simulink model "induction_foc"  (R2022b)
settings: Solver=ode15s  StartTime=0.0  StopTime=2  MaxStep=1e-4  MinStep=1e-7  RelTol=1e-3
values from neighbouring files (symbols this model uses):
  al = log(9)/tr_m    [parameters_4.m]
  as = log(9)/tr_s    [parameters_4.m]
  ba = 2 * K^2 * (as * J)/(3*np^2 * psi_nom)    [parameters_4.m]
  I_base = 3.6 * sqrt(2)    [parameters_4.m]
  Id_nom = psi_nom/LM    [parameters_4.m]
  J = 0.1    [parameters_4.m]
  J_m = J    (= 0.1)    [parameters_4.m]
  K = 1    [parameters_4.m]
  Ki = (ac^2)*Lsig    [parameters_4.m]
  Kis = 2*K^2 * as^2 * J/(3*np^2 * psi_nom)    [parameters_4.m]
  Kp = ac*Lsig    [parameters_4.m]
  Kps = 2*K^2 * as * J/(3*np^2 * psi_nom)    [parameters_4.m]
  ksi = (Lsig + LM)/Lsig    (= 10.2245098039)    [parameters_4.m]
  lamba = 1.5    [parameters_4.m]
  LM = b*Lm    (= 0.368980392157)    [parameters_4.m]
  LM_m = LM    (= 0.368980392157)    [parameters_4.m]
  LMest = LMest2    (= 0.368980392157)    [parameters_4.m]
  LMest2 = LM    (= 0.368980392157)    [parameters_4.m]
  Lsig = Lls+Llr    (= 0.04)    [parameters_4.m]
  Lsig_m = Lsig    (= 0.04)    [parameters_4.m]
  np = 2    [parameters_4.m]
  Ra = ac*Lsig-Rs-RR    [parameters_4.m]
  RR = (b^2)*Rr    (= 2.26090926567)    [parameters_4.m]
  RR_m = RR    (= 2.26090926567)    [parameters_4.m]
  RRest = RRest2    (= 2.26090926567)    [parameters_4.m]
  RRest2 = RR    (= 2.26090926567)    [parameters_4.m]
  Rs = 6.5    [parameters_4.m]
  Rs_m = Rs    (= 6.5)    [parameters_4.m]
  V_base = 60    [parameters_4.m]
  Vpeak = V_base    (= 60)    [parameters_4.m]
  w_base = 2*pi*50    (= 314.159265359)    [parameters_4.m]
  w_delta = 0.1*w_base    (= 31.4159265359)    [parameters_4.m]
undefined symbols (not defined in the file or in its folder): I_max, sigbuilder_block
libraries: simulink x2
settings Model: Creator=alexa  LastModifiedBy=alexa
settings SolverCC: InitialStep=1e-6

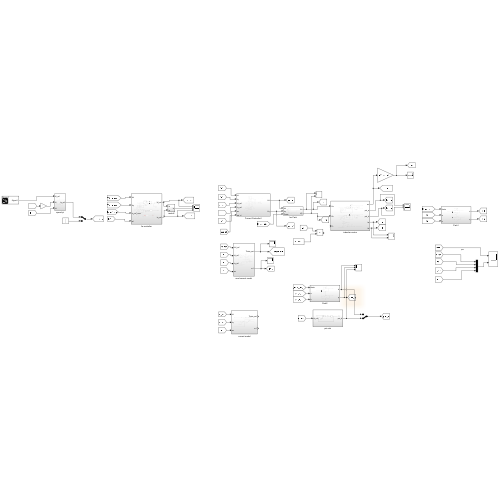
[thumbnail: Simulink's stored preview of the top-level diagram]
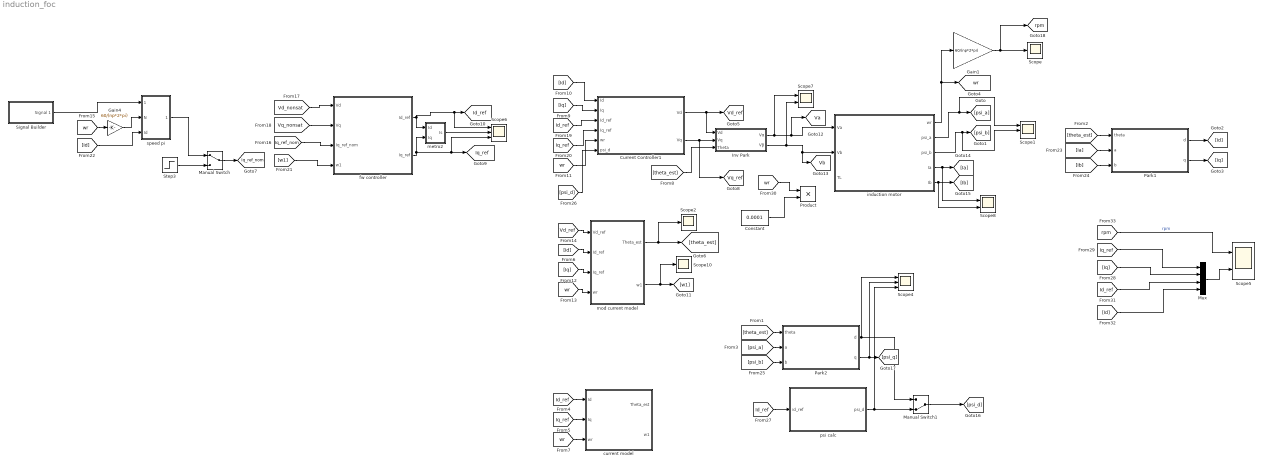
== system induction_foc ==
  Constant : Constant  Value=0.0001
  Current Controller1 : Subsystem
  Gain1 : Gain  Gain=60/(np*2*pi)
  Gain4 : Gain  Gain=60/(np*2*pi)
  Inv Park : Subsystem
  Manual Switch : ManualSwitch
  Manual Switch1 : ManualSwitch  CurrentSetting=0
  Mux : Mux
  Park1 : Subsystem
  Park2 : Subsystem
  Product : Product
  Scope : Scope
  Scope1 : Scope  NumInputPorts=3
  Scope10 : Scope
  Scope2 : Scope
  Scope4 : Scope  NumInputPorts=3
  Scope5 : Scope  NumInputPorts=2
  Scope6 : Scope  NumInputPorts=3
  Scope7 : Scope  NumInputPorts=2
  Scope8 : Scope  NumInputPorts=2
  Signal Builder : Subsystem  Tag=STV Subsys  LoadFcn=sigbuilder_block('load');  StartFcn=sigbuilder_block('start');  StopFcn=sigbuilder_block('stop');  ClipboardFcn=sigbuilder_block('clipboard');  mask(Sigbuilder block){tuvar=[0:10]}
      mask help: Simulink:masks:SigbuilderBlock_MD
      mask init:
      | if ~strcmp(get_param(bdroot(gcbh),'SimulationStatus'),'stopped') tuvar = sigbuilder_block('maskInit'); end
      settings: CopyFcn=sigbuilder_block('copy');  DeleteFcn=sigbuilder_block('delete');  ModelCloseFcn=sigbuilder_block('modelClose');  PreSaveFcn=sigbuilder_block('preSave');  PauseFcn=sigbuilder_block('pause');  ContinueFcn=sigbuilder_block('continue');  NameChangeFcn=sigbuilder_block('namechange');  OpenFcn=sigbuilder_block('open',[437.6 199.2 550.4 400 ]);  CloseFcn=sigbuilder_block('close');
      mask Display: plot(0, 0, 100, 100,[2, 2, 32, 32, 2], [68, 8, 8, 68, 68],[32, 2], [38, 38], [32, 19, 2],[53, 60, 44], [32, 17, 17, 2],[16, 16, 31, 31]);txt = getActiveGroup(gcbh);text(2, 100, txt,'verticalAlignment', 'top');
  Step3 : Step  Time=0.3  After=3  SampleTime=0
  current model : Subsystem
  fw controller : Subsystem
  induction motor : Subsystem
  metro2 : Subsystem
  mod current model : Subsystem
  psi calc : Subsystem
  speed pi : Subsystem
  tag scope: Id_ref=global, Iq_ref=global, Iq_ref_nom=global, Va=global, Vb=global, Vd_ref=global, Vq_ref=global, rpm=global, wr=global
  wires:
  Inv Park/1(Vα) -> Scope7/1, [Va], induction motor/1(Va)
  Inv Park/2(Vβ) -> Scope7/2, [Vb], induction motor/2(Vb)
  induction motor/1(wr) -> Gain1/1, [wr]
  induction motor/2(psi_a) -> Scope1/1, [psi_a]
  induction motor/3(psi_b) -> Scope1/2, [psi_b]
  [theta_est] -> Park1/1(theta)
  Park1/1(d) -> [Id]
  Park1/2(q) -> [Iq]
  Current Controller1/2(Vq) -> [Vq_ref], Inv Park/2(Vq)
  Current Controller1/1(Vd) -> [Vd_ref], Inv Park/1(Vd)
  [theta_est] -> Inv Park/3(Theta)
  [Id_ref] -> Current Controller1/3(Id_ref)
  [Iq] -> Current Controller1/2(Iq)
  [Id] -> Current Controller1/1(Id)
  [wr] -> Current Controller1/5(wr)
  Gain4/1 -> speed pi/2(N)
  Signal Builder/1(Signal 1) -> speed pi/1(N_ref)
  [Id_ref] -> current model/1(Id)
  [wr] -> current model/3(wr)
  [Iq_ref] -> current model/2(Iq)
  [Iq] -> mod current model/3(Iq_ref)
  [Id] -> mod current model/2(Id_ref)
  [wr] -> mod current model/4(wr)
  [Vd_ref] -> mod current model/1(Vd_ref)
  [wr] -> Gain4/1
  [Vd_nonsat] -> fw controller/1(Vd)
  [Vq_nonsat] -> fw controller/2(Vq)
  [Iq_ref] -> Current Controller1/4(Iq_ref)
  fw controller/2(Iq_ref) -> metro2/2(Iq), Scope6/3, [Iq_ref]
  fw controller/1(Id_ref) -> Scope6/1, [Id_ref], metro2/1(Id)
  [w1] -> fw controller/4(w1)
  Gain1/1 -> [rpm], Scope/1
  metro2/1(Is) -> Scope6/2
  [Iq_ref_nom] -> fw controller/3(Iq_ref_nom)
  [Id] -> speed pi/3(Id)
  mod current model/1(Theta_est) -> Scope2/1, [theta_est]
  mod current model/2(w1) -> Scope10/1, [w1]
  induction motor/4(Ia) -> Scope8/1, [Ia]
  induction motor/5(Ib) -> Scope8/2, [Ib]
  [Ib] -> Park1/3(b)
  [Ia] -> Park1/2(a)
  [theta_est] -> Park2/1(theta)
  [psi_a] -> Park2/2(a)
  [psi_b] -> Park2/3(b)
  Park2/1(d) -> Scope4/1, Manual Switch1/1
  Park2/2(q) -> Scope4/2, [psi_q]
  [psi_d] -> Current Controller1/6(psi_d)
  psi calc/1(psi_d) -> Manual Switch1/2, Scope4/3
  [Id_ref] -> psi calc/1(id_ref)
  [wr] -> Product/1
  Constant/1 -> Product/2
  Step3/1 -> Manual Switch/2
  speed pi/1(Iq_ref) -> Manual Switch/1
  Manual Switch/1 -> [Iq_ref_nom]
  Manual Switch1/1 -> [psi_d]
  [Iq_ref] -> Mux/1
  [Iq] -> Mux/2
  [Id_ref] -> Mux/3
  [Id] -> Mux/4
  Mux/1 -> Scope5/2
  [rpm] -> Scope5/1  "rpm"

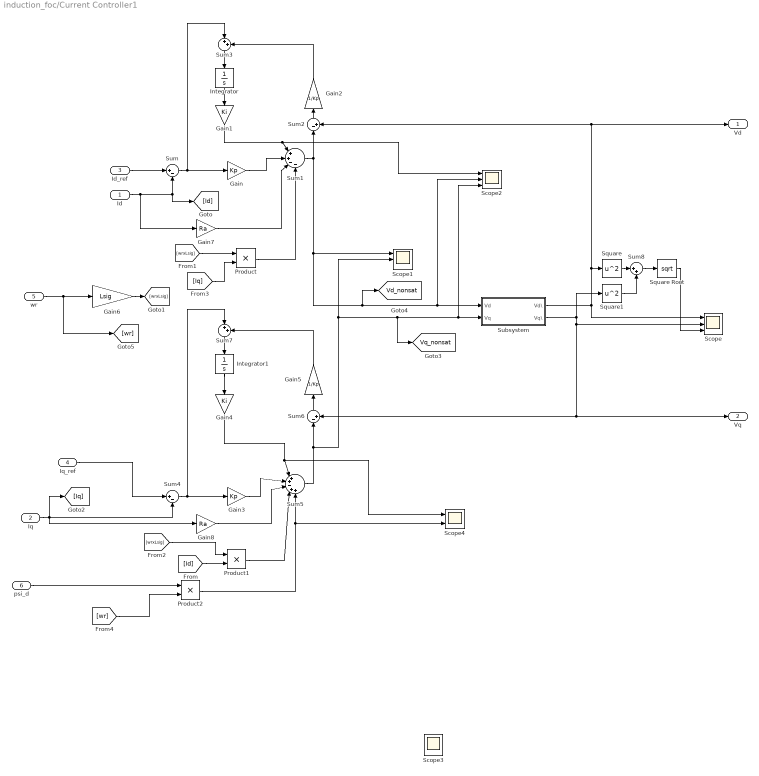
== system induction_foc/Current Controller1 ==
  Id : Inport
  Iq : Inport  Port=2
  Id_ref : Inport  Port=3
  Iq_ref : Inport  Port=4
  wr : Inport  Port=5
  psi_d : Inport  Port=6
  Gain : Gain  Gain=Kp
  Gain1 : Gain  Gain=Ki
  Gain2 : Gain  Gain=1/Kp
  Gain3 : Gain  Gain=Kp
  Gain4 : Gain  Gain=Ki
  Gain5 : Gain  Gain=1/Kp
  Gain6 : Gain  Gain=Lsig
  Gain7 : Gain  Gain=Ra
  Gain8 : Gain  Gain=Ra
  Integrator : Integrator
  Integrator1 : Integrator
  Product : Product
  Product1 : Product
  Product2 : Product
  Scope{,1..3} (4 alike) : Scope  NumInputPorts=3
  Scope4 : Scope  NumInputPorts=2
  Square : Math  Operator=square
  Square Root : Sqrt
  Square1 : Math  Operator=square
  Subsystem : Subsystem
  Sum : Sum  Inputs=|+-
  Sum1 : Sum  Inputs=|++--
  Sum2 : Sum  Inputs=|-+
  Sum3 : Sum  Inputs=|++
  Sum4 : Sum  Inputs=|+-
  Sum5 : Sum  Inputs=|++-++
  Sum6 : Sum  Inputs=|-+
  Sum7 : Sum  Inputs=|++
  Sum8 : Sum  Inputs=|++
  Vd : Outport
  Vq : Outport  Port=2
  tag scope: Vd_nonsat=global, Vq_nonsat=global
  wires:
  Id_ref/1 -> Sum/1
  Id/1 -> Gain7/1, [Id], Sum/2
  Sum/1 -> Sum3/1, Gain/1
  Subsystem/1(Vd\) -> Square/1, Sum2/2, Vd/1, Scope/1
  Integrator/1 -> Gain1/1
  Sum3/1 -> Integrator/1
  Sum2/1 -> Gain2/1
  Gain/1 -> Sum1/2
  Gain1/1 -> Scope2/1, Sum1/1
  Gain5/1 -> Sum7/2
  Integrator1/1 -> Gain4/1
  Sum4/1 -> Sum7/1, Gain3/1
  Subsystem/2(Vq\) -> Scope/2, Sum6/2, Vq/1, Square1/1
  Gain3/1 -> Sum5/2
  Gain4/1 -> Scope4/1, Sum5/1
  Sum7/1 -> Integrator1/1
  Iq_ref/1 -> Sum4/1
  Sum6/1 -> Gain5/1
  Sum5/1 -> Sum6/1, [Vq_nonsat], Scope2/3, Subsystem/2(Vq), Scope1/2
  Iq/1 -> Gain8/1, Sum4/2, [Iq]
  wr/1 -> [wr], Gain6/1
  Product/1 -> Sum1/4
  [Id] -> Product1/2
  Gain6/1 -> [wrxLsig]
  [wrxLsig] -> Product/1
  [wrxLsig] -> Product1/1
  Product1/1 -> Sum5/4
  [Iq] -> Product/2
  Gain7/1 -> Sum1/3
  Gain8/1 -> Sum5/3
  Gain2/1 -> Sum3/2
  Square/1 -> Sum8/1
  Square1/1 -> Sum8/2
  Sum8/1 -> Square Root/1
  Square Root/1 -> Scope/3
  Sum1/1 -> [Vd_nonsat], Scope2/2, Subsystem/1(Vd), Scope1/1, Sum2/1
  psi_d/1 -> Product2/1
  [wr] -> Product2/2
  Product2/1 -> Scope4/2, Sum5/5

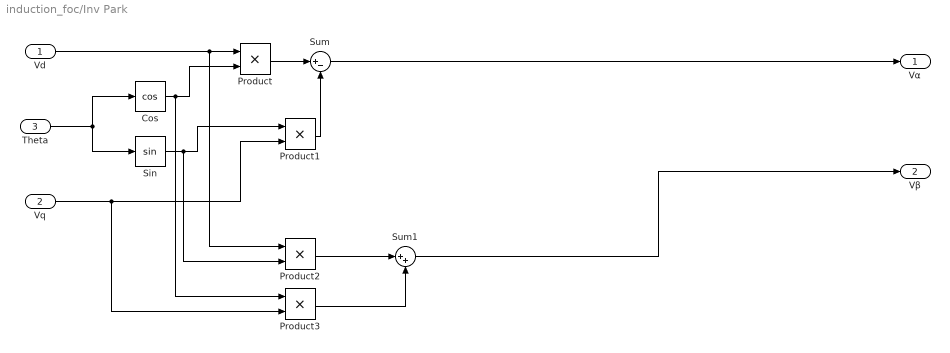
== system induction_foc/Inv Park ==
  Vd : Inport
  Vq : Inport  Port=2
  Theta : Inport  Port=3
  Cos : Trigonometry  Operator=cos
  Product{,1..3} (4 alike) : Product
  Sin : Trigonometry
  Sum : Sum  Inputs=|+-
  Sum1 : Sum  Inputs=|++
  Vα : Outport
  Vβ : Outport  Port=2
  wires:
  Theta/1 -> Sin/1, Cos/1
  Vd/1 -> Product2/1, Product/1
  Cos/1 -> Product3/1, Product/2
  Product/1 -> Sum/1
  Sin/1 -> Product2/2, Product1/1
  Vq/1 -> Product3/2, Product1/2
  Product1/1 -> Sum/2
  Sum/1 -> Vα/1
  Product2/1 -> Sum1/1
  Product3/1 -> Sum1/2
  Sum1/1 -> Vβ/1

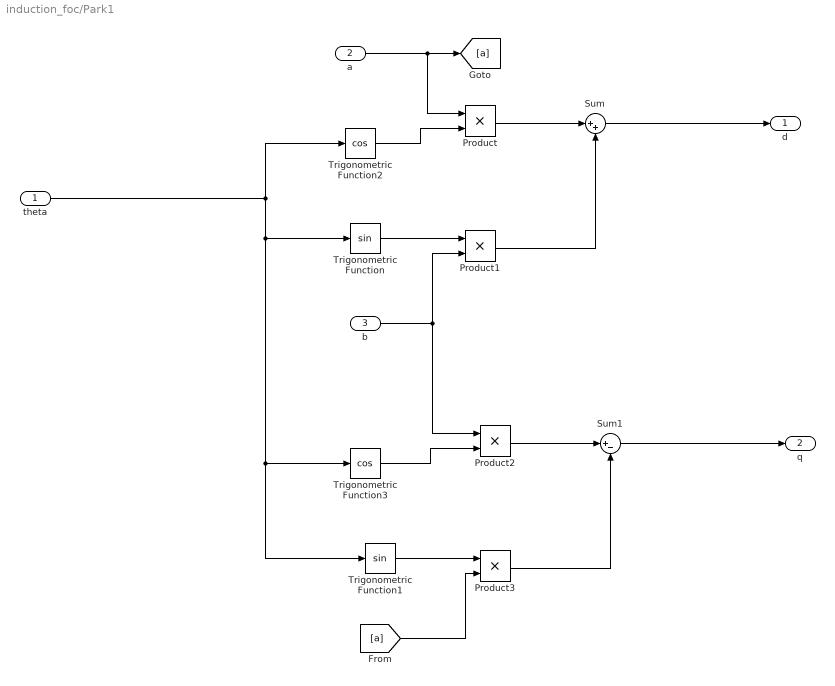
== system induction_foc/Park1 ==
  theta : Inport
  a : Inport  Port=2
  b : Inport  Port=3
  Product{,1..3} (4 alike) : Product
  Sum : Sum  Inputs=|++
  Sum1 : Sum  Inputs=|+-
  Trigonometric Function : Trigonometry
  Trigonometric Function1 : Trigonometry
  Trigonometric Function2 : Trigonometry  Operator=cos
  Trigonometric Function3 : Trigonometry  Operator=cos
  d : Outport
  q : Outport  Port=2
  wires:
  Trigonometric Function2/1 -> Product/2
  a/1 -> [a], Product/1
  Product/1 -> Sum/1
  Trigonometric Function/1 -> Product1/1
  b/1 -> Product1/2, Product2/1
  Product1/1 -> Sum/2
  Sum/1 -> d/1
  Trigonometric Function3/1 -> Product2/2
  Trigonometric Function1/1 -> Product3/1
  Sum1/1 -> q/1
  Product2/1 -> Sum1/1
  Product3/1 -> Sum1/2
  [a] -> Product3/2
  theta/1 -> Trigonometric Function/1, Trigonometric Function3/1, Trigonometric Function1/1, Trigonometric Function2/1

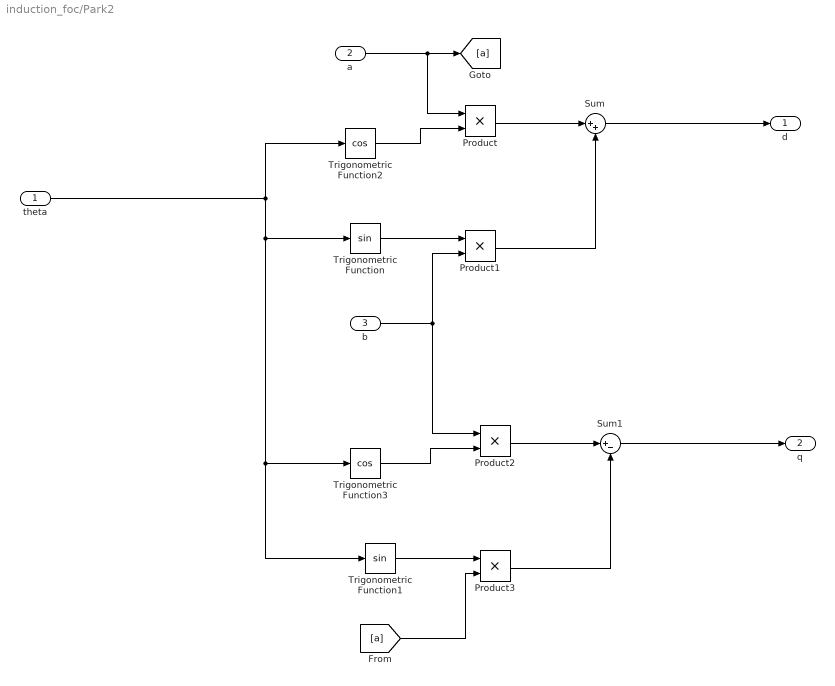
== system induction_foc/Park2 ==
  theta : Inport
  a : Inport  Port=2
  b : Inport  Port=3
  Product{,1..3} (4 alike) : Product
  Sum : Sum  Inputs=|++
  Sum1 : Sum  Inputs=|+-
  Trigonometric Function : Trigonometry
  Trigonometric Function1 : Trigonometry
  Trigonometric Function2 : Trigonometry  Operator=cos
  Trigonometric Function3 : Trigonometry  Operator=cos
  d : Outport
  q : Outport  Port=2
  wires:
  Trigonometric Function2/1 -> Product/2
  a/1 -> [a], Product/1
  Product/1 -> Sum/1
  Trigonometric Function/1 -> Product1/1
  b/1 -> Product1/2, Product2/1
  Product1/1 -> Sum/2
  Sum/1 -> d/1
  Trigonometric Function3/1 -> Product2/2
  Trigonometric Function1/1 -> Product3/1
  Sum1/1 -> q/1
  Product2/1 -> Sum1/1
  Product3/1 -> Sum1/2
  [a] -> Product3/2
  theta/1 -> Trigonometric Function/1, Trigonometric Function3/1, Trigonometric Function1/1, Trigonometric Function2/1

== system induction_foc/Signal Builder ==
  Demux : Demux  Tag=STV Demux  Outputs=1
      settings: DisplayOption=none
  FromWs : FromWorkspace  Tag=STV FromWs  VariableName=tuvar
      SigBuilderData=|
      | common.afterFinalStr = 'Extrapolate'
      | common.sampleTime = 0
      | dataSet.timeRange = [0 10]
      | dataSet.name = 'Group 1'
      | sbobj.Groups.Name = 'Group 1'
      | sbobj.Groups.Signals.Name = 'Signal 1'
      | sbobj.Groups.Signals.XData = [0 0.5 0.5 1 1 10]
      | sbobj.Groups.Signals.YData = [0 52 200 200 0 0]
  Signal 1 : Outport  Tag=STV Outport
  wires:
  Demux/1 -> Signal 1/1
  FromWs/1 -> Demux/1

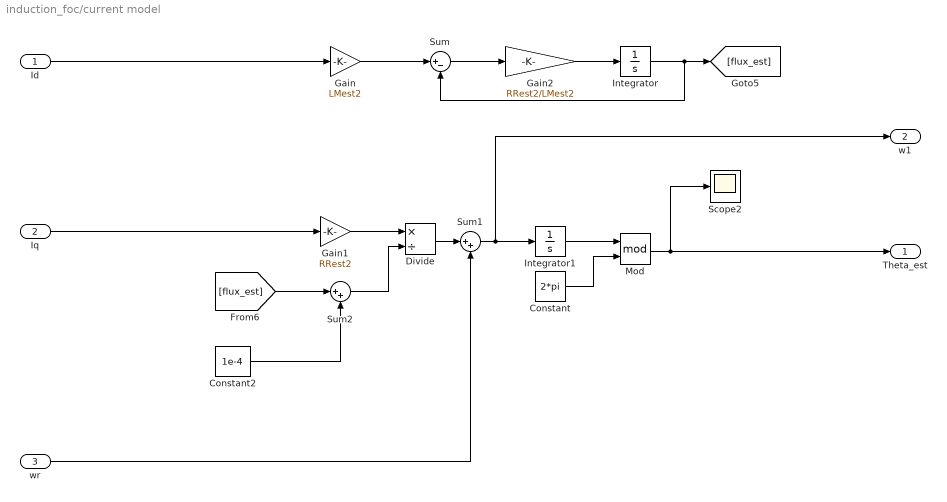
== system induction_foc/current model ==
  Id : Inport
  Iq : Inport  Port=2
  wr : Inport  Port=3
  Constant : Constant  Value=2*pi
  Constant2 : Constant  Value=1e-4
  Divide : Product  Inputs=*/
  Gain : Gain  Gain=LMest2
  Gain1 : Gain  Gain=RRest2
  Gain2 : Gain  Gain=RRest2/LMest2
  Integrator : Integrator
  Integrator1 : Integrator
  Mod : Math  Operator=mod
  Scope2 : Scope
  Sum : Sum  Inputs=|+-
  Sum1 : Sum  Inputs=|++
  Sum2 : Sum  Inputs=|++
  Theta_est : Outport
  w1 : Outport  Port=2
  wires:
  Sum2/1 -> Divide/2
  Constant/1 -> Mod/2
  Integrator/1 -> Sum/2, [flux_est]
  Divide/1 -> Sum1/1
  Gain/1 -> Sum/1
  [flux_est] -> Sum2/1
  Constant2/1 -> Sum2/2
  Sum1/1 -> w1/1, Integrator1/1
  wr/1 -> Sum1/2
  Gain1/1 -> Divide/1
  Gain2/1 -> Integrator/1
  Id/1 -> Gain/1
  Sum/1 -> Gain2/1
  Mod/1 -> Theta_est/1, Scope2/1
  Iq/1 -> Gain1/1
  Integrator1/1 -> Mod/1

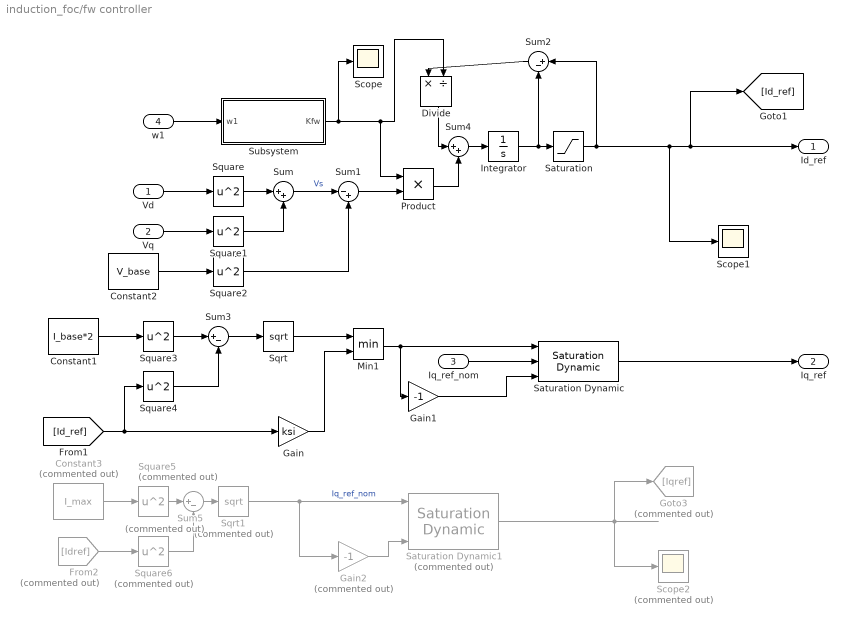
== system induction_foc/fw controller ==
  Vd : Inport
  Vq : Inport  Port=2
  Iq_ref_nom : Inport  Port=3
  w1 : Inport  Port=4
  Constant1 : Constant  Value=I_base*2
  Constant2 : Constant  Value=V_base
  Constant3 : Constant  Commented=on  Value=I_max
  Divide : Product  Inputs=*/
  From2 : From  Commented=on  GotoTag=Idref
  Gain : Gain  Gain=ksi
  Gain1 : Gain  Gain=-1
  Gain2 : Gain  Commented=on  Gain=-1
  Goto3 : Goto  Commented=on  GotoTag=Iqref
  Integrator : Integrator
  Min1 : MinMax  Inputs=2
  Product : Product
  Saturation : Saturate  UpperLimit=Id_nom  LowerLimit=0.05*Id_nom
  Saturation Dynamic : simulink/Discontinuities/Saturation Dynamic  OutMin=[]  OutMax=[]  OutDataTypeStr=Inherit: Same as second input  OutDataType=fixdt(1, 16)  OutScaling=2^-10  DoSatur=off
  Saturation Dynamic1 : simulink/Discontinuities/Saturation Dynamic  Commented=on  OutMin=[]  OutMax=[]  OutDataTypeStr=Inherit: Same as second input  OutDataType=fixdt(1, 16)  OutScaling=2^-10  DoSatur=off
  Scope : Scope
  Scope1 : Scope
  Scope2 : Scope  Commented=on
  Sqrt : Sqrt
  Sqrt1 : Sqrt  Commented=on
  Square{,1..4} (5 alike) : Math  Operator=square
  Square5 : Math  Commented=on  Operator=square
  Square6 : Math  Commented=on  Operator=square
  Subsystem : Subsystem
  Sum : Sum  Inputs=|++
  Sum1 : Sum  Inputs=|-+
  Sum2 : Sum  Inputs=|+-
  Sum3 : Sum  Inputs=|+-
  Sum4 : Sum  Inputs=|++
  Sum5 : Sum  Commented=on  Inputs=|+-
  Id_ref : Outport
  Iq_ref : Outport  Port=2
  wires:
  Vd/1 -> Square/1
  Vq/1 -> Square1/1
  Constant2/1 -> Square2/1
  Square/1 -> Sum/1
  Square1/1 -> Sum/2
  Sum/1 -> Sum1/1  "Vs"
  Square2/1 -> Sum1/2
  Sum1/1 -> Product/2
  Integrator/1 -> Sum2/2, Saturation/1
  w1/1 -> Subsystem/1(w1)
  Subsystem/1(Kfw) -> Scope/1, Divide/2, Product/1
  Constant1/1 -> Square3/1
  Square3/1 -> Sum3/1
  Square4/1 -> Sum3/2
  Sum3/1 -> Sqrt/1
  Sqrt/1 -> Min1/1
  Gain/1 -> Min1/2
  [Id_ref] -> Square4/1, Gain/1
  Iq_ref_nom/1 -> Saturation Dynamic/2
  Min1/1 -> Gain1/1, Saturation Dynamic/1
  Gain1/1 -> Saturation Dynamic/3
  Saturation Dynamic/1 -> Iq_ref/1
  Saturation/1 -> Sum2/1, Scope1/1, [Id_ref], Id_ref/1
  Product/1 -> Sum4/2
  Sum4/1 -> Integrator/1
  Sum2/1 -> Divide/1
  Divide/1 -> Sum4/1
  ? -> Saturation Dynamic1/2
  Sum5/1 -> Sqrt1/1
  Square6/1 -> Sum5/2
  From2/1 -> Square6/1
  Saturation Dynamic1/1 -> Scope2/1, Goto3/1
  Square5/1 -> Sum5/1
  Sqrt1/1 -> Saturation Dynamic1/1, Gain2/1  "Iq_ref_nom"
  Constant3/1 -> Square5/1
  Gain2/1 -> Saturation Dynamic1/3

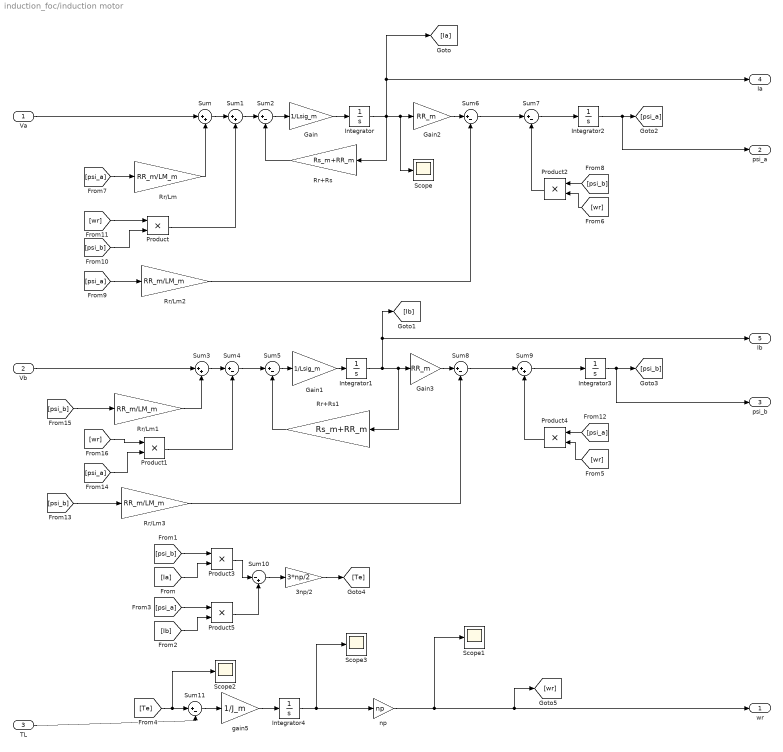
== system induction_foc/induction motor ==
  Va : Inport
  Vb : Inport  Port=2
  TL : Inport  Port=3
  3np/2 : Gain  Gain=3*np/2
  Gain : Gain  Gain=1/Lsig_m
  Gain1 : Gain  Gain=1/Lsig_m
  Gain2 : Gain  Gain=RR_m
  Gain3 : Gain  Gain=RR_m
  Integrator{,1..4} (5 alike) : Integrator
  Product{,1..5} (6 alike) : Product
  Rr+Rs : Gain  Gain=Rs_m+RR_m
  Rr+Rs1 : Gain  Gain=Rs_m+RR_m
  Rr/Lm{,1..3} (4 alike) : Gain  Gain=RR_m/LM_m
  Scope{,1..3} (4 alike) : Scope
  Sum{,1,3,9} (4 alike) : Sum  Inputs=|++
  Sum10 : Sum  Inputs=|-+
  Sum{2,4..8,11} (7 alike) : Sum  Inputs=|+-
  gain5 : Gain  Gain=1/J_m
  np : Gain  Gain=np
  wr : Outport
  psi_a : Outport  Port=2
  psi_b : Outport  Port=3
  Ia : Outport  Port=4
  Ib : Outport  Port=5
  wires:
  Va/1 -> Sum/1
  Sum/1 -> Sum1/1
  Rr/Lm/1 -> Sum/2
  Integrator2/1 -> psi_a/1, [psi_a]
  Product/1 -> Sum1/2
  Rr+Rs/1 -> Sum2/2
  Integrator/1 -> Scope/1, Gain2/1, Ia/1, [Ia], Rr+Rs/1
  Sum1/1 -> Sum2/1
  Sum2/1 -> Gain/1
  Gain/1 -> Integrator/1
  Integrator3/1 -> psi_b/1, [psi_b]
  Gain1/1 -> Integrator1/1
  Sum4/1 -> Sum5/1
  Integrator1/1 -> Rr+Rs1/1, Gain3/1, [Ib], Ib/1
  Sum5/1 -> Gain1/1
  Vb/1 -> Sum3/1
  Sum3/1 -> Sum4/1
  Rr+Rs1/1 -> Sum5/2
  Product1/1 -> Sum4/2
  Gain2/1 -> Sum6/1
  Rr/Lm2/1 -> Sum6/2
  Sum6/1 -> Sum7/1
  Product2/1 -> Sum7/2
  Sum7/1 -> Integrator2/1
  Rr/Lm3/1 -> Sum8/2
  Product4/1 -> Sum9/2
  Sum8/1 -> Sum9/1
  Sum9/1 -> Integrator3/1
  Gain3/1 -> Sum8/1
  [psi_b] -> Product3/1
  [Ia] -> Product3/2
  [psi_a] -> Product5/1
  [Ib] -> Product5/2
  Product3/1 -> Sum10/1
  Product5/1 -> Sum10/2
  Sum10/1 -> 3np/2/1
  3np/2/1 -> [Te]
  [Te] -> Scope2/1, Sum11/1
  Sum11/1 -> gain5/1
  gain5/1 -> Integrator4/1
  TL/1 -> Sum11/2
  [wr] -> Product4/2
  np/1 -> Scope1/1, [wr], wr/1
  [psi_a] -> Rr/Lm/1
  [psi_b] -> Product2/1
  [wr] -> Product2/2
  [psi_a] -> Rr/Lm2/1
  [psi_b] -> Product/2
  [wr] -> Product/1
  [psi_a] -> Product4/1
  [psi_a] -> Product1/2
  [psi_b] -> Rr/Lm1/1
  [wr] -> Product1/1
  Integrator4/1 -> Scope3/1, np/1
  Rr/Lm1/1 -> Sum3/2
  [psi_b] -> Rr/Lm3/1

== system induction_foc/metro2 ==
  Id : Inport
  Iq : Inport  Port=2
  Sqrt : Sqrt
  Square : Math  Operator=square
  Square1 : Math  Operator=square
  Sum : Sum  Inputs=|++
  Is : Outport
  wires:
  Id/1 -> Square/1
  Iq/1 -> Square1/1
  Square/1 -> Sum/1
  Square1/1 -> Sum/2
  Sum/1 -> Sqrt/1
  Sqrt/1 -> Is/1

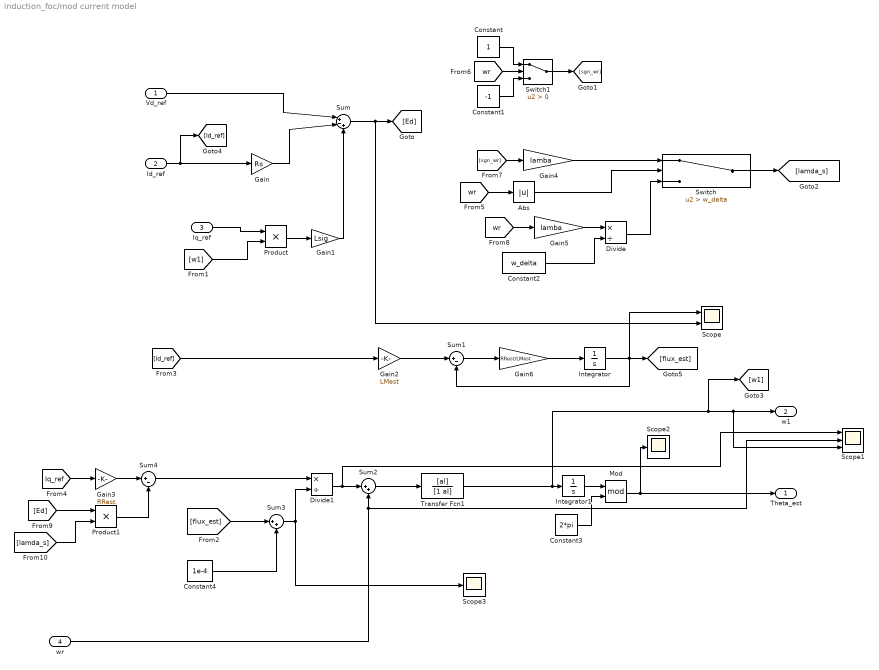
== system induction_foc/mod current model ==
  Vd_ref : Inport
  Id_ref : Inport  Port=2
  Iq_ref : Inport  Port=3
  wr : Inport  Port=4
  Abs : Abs  SaturateOnIntegerOverflow=off
  Constant : Constant
  Constant1 : Constant  Value=-1
  Constant2 : Constant  Value=w_delta
  Constant3 : Constant  Value=2*pi
  Constant4 : Constant  Value=1e-4
  Divide : Product  Inputs=*/
  Divide1 : Product  Inputs=*/
  Gain : Gain  Gain=Rs
  Gain1 : Gain  Gain=Lsig
  Gain2 : Gain  Gain=LMest
  Gain3 : Gain  Gain=RRest
  Gain4 : Gain  Gain=lamba
  Gain5 : Gain  Gain=lamba
  Gain6 : Gain  Gain=RRest/LMest
  Integrator : Integrator
  Integrator1 : Integrator
  Mod : Math  Operator=mod
  Product : Product
  Product1 : Product
  Scope : Scope  NumInputPorts=2
  Scope1 : Scope  NumInputPorts=3
  Scope2 : Scope
  Scope3 : Scope
  Sum : Sum  Inputs=|+-+
  Sum1 : Sum  Inputs=|+-
  Sum2 : Sum  Inputs=|++
  Sum3 : Sum  Inputs=|++
  Sum4 : Sum  Inputs=|+-
  Switch : Switch  Criteria=u2 > Threshold  Threshold=w_delta  SaturateOnIntegerOverflow=off  InputSameDT=off
  Switch1 : Switch  Criteria=u2 > Threshold  SaturateOnIntegerOverflow=off  InputSameDT=off
  Transfer Fcn1 : TransferFcn  Numerator=[al]  Denominator=[1 al]
  Theta_est : Outport
  w1 : Outport  Port=2
  wires:
  Vd_ref/1 -> Sum/1
  Gain/1 -> Sum/2
  [w1] -> Product/2
  Product/1 -> Gain1/1
  Gain1/1 -> Sum/3
  Sum/1 -> Scope/2, [Ed]
  [wr] -> Abs/1
  Abs/1 -> Switch/2
  [wr] -> Switch1/2
  Constant/1 -> Switch1/1
  Constant1/1 -> Switch1/3
  Switch1/1 -> [sgn_wr]
  [sgn_wr] -> Gain4/1
  Gain4/1 -> Switch/1
  [wr] -> Gain5/1
  Gain5/1 -> Divide/1
  Constant2/1 -> Divide/2
  Divide/1 -> Switch/3
  Switch/1 -> [lamda_s]
  Id_ref/1 -> [Id_ref], Gain/1
  Iq_ref/1 -> Product/1
  Constant4/1 -> Sum3/2
  wr/1 -> Scope1/2, Sum2/2
  [flux_est] -> Sum3/1
  Gain6/1 -> Integrator/1
  Sum1/1 -> Gain6/1
  Integrator1/1 -> Mod/1
  Gain2/1 -> Sum1/1
  Mod/1 -> Scope2/1, Theta_est/1
  Divide1/1 -> Scope1/1, Sum2/1
  [Id_ref] -> Gain2/1
  Integrator/1 -> Sum1/2, Scope/1, [flux_est]
  Constant3/1 -> Mod/2
  Sum3/1 -> Divide1/2, Scope3/1
  [Iq_ref] -> Gain3/1
  Gain3/1 -> Sum4/1
  Sum4/1 -> Divide1/1
  Product1/1 -> Sum4/2
  [Ed] -> Product1/1
  [lamda_s] -> Product1/2
  Sum2/1 -> Transfer Fcn1/1
  Transfer Fcn1/1 -> [w1], Scope1/3, w1/1, Integrator1/1

== system induction_foc/psi calc ==
  id_ref : Inport
  Add : Sum  Inputs=+-
  Gain : Gain  Gain=1/LM
  Gain1 : Gain  Gain=RR
  Integrator : Integrator
  psi_d : Outport
  wires:
  id_ref/1 -> Add/1
  Add/1 -> Gain1/1
  Gain/1 -> Add/2
  Integrator/1 -> psi_d/1, Gain/1
  Gain1/1 -> Integrator/1

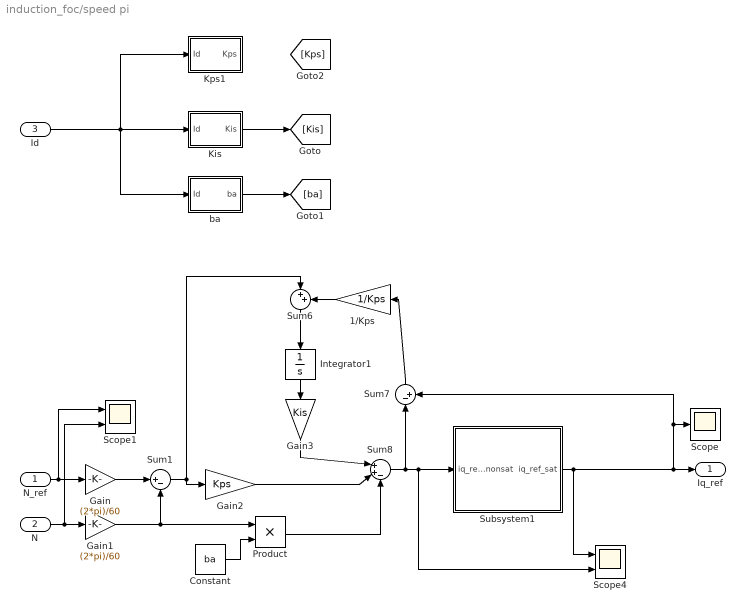
== system induction_foc/speed pi ==
  N_ref : Inport
  N : Inport  Port=2
  Id : Inport  Port=3
  1/Kps : Gain  Gain=1/Kps
  Constant : Constant  Value=ba
  Gain : Gain  Gain=(2*pi)/60
  Gain1 : Gain  Gain=(2*pi)/60
  Gain2 : Gain  Gain=Kps
  Gain3 : Gain  Gain=Kis
  Integrator1 : Integrator
  Kis : Subsystem
  Kps1 : Subsystem
  Product : Product
  Scope : Scope
  Scope1 : Scope  NumInputPorts=2
  Scope4 : Scope  NumInputPorts=2
  Subsystem1 : Subsystem
  Sum1 : Sum  Inputs=|+-
  Sum6 : Sum  Inputs=|++
  Sum7 : Sum  Inputs=|-+
  Sum8 : Sum  Inputs=|++-
  ba : Subsystem
  Iq_ref : Outport
  wires:
  Subsystem1/1(iq_ref_sat) -> Scope4/1, Sum7/2, Scope/1, Iq_ref/1
  Sum7/1 -> 1/Kps/1
  Sum8/1 -> Scope4/2, Subsystem1/1(iq_ref_nonsat), Sum7/1
  Gain2/1 -> Sum8/2
  1/Kps/1 -> Sum6/2
  Sum1/1 -> Gain2/1, Sum6/1
  N_ref/1 -> Scope1/1, Gain/1
  N/1 -> Scope1/2, Gain1/1
  Constant/1 -> Product/2
  Sum6/1 -> Integrator1/1
  Gain3/1 -> Sum8/1
  Product/1 -> Sum8/3
  Gain/1 -> Sum1/1
  Gain1/1 -> Product/1, Sum1/2
  Id/1 -> Kps1/1(Id), ba/1(Id), Kis/1(Id)
  Kis/1(Kis) -> [Kis]
  ba/1(ba) -> [ba]
  Integrator1/1 -> Gain3/1

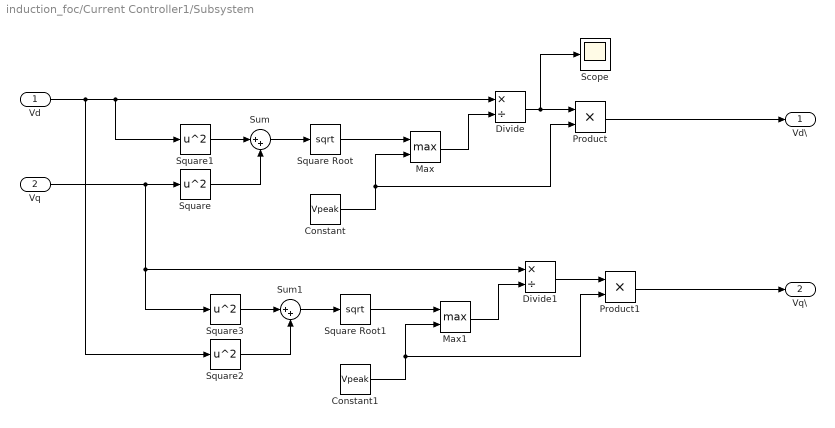
== system induction_foc/Current Controller1/Subsystem ==
  Vd : Inport
  Vq : Inport  Port=2
  Constant : Constant  Value=Vpeak
  Constant1 : Constant  Value=Vpeak
  Divide : Product  Inputs=*/
  Divide1 : Product  Inputs=*/
  Max : MinMax  Function=max  Inputs=2
  Max1 : MinMax  Function=max  Inputs=2
  Product : Product
  Product1 : Product
  Scope : Scope
  Square{,1..3} (4 alike) : Math  Operator=square
  Square Root : Sqrt
  Square Root1 : Sqrt
  Sum : Sum  Inputs=|++
  Sum1 : Sum  Inputs=|++
  Vd\ : Outport
  Vq\ : Outport  Port=2
  wires:
  Square1/1 -> Sum/1
  Square/1 -> Sum/2
  Sum/1 -> Square Root/1
  Square Root/1 -> Max/1
  Constant/1 -> Product/2, Max/2
  Max/1 -> Divide/2
  Divide/1 -> Scope/1, Product/1
  Product/1 -> Vd\/1
  Square3/1 -> Sum1/1
  Constant1/1 -> Product1/2, Max1/2
  Square2/1 -> Sum1/2
  Divide1/1 -> Product1/1
  Vd/1 -> Square2/1, Divide/1, Square1/1
  Vq/1 -> Divide1/1, Square3/1, Square/1
  Square Root1/1 -> Max1/1
  Max1/1 -> Divide1/2
  Sum1/1 -> Square Root1/1
  Product1/1 -> Vq\/1

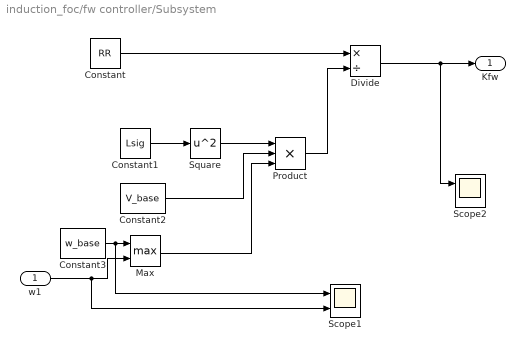
== system induction_foc/fw controller/Subsystem ==
  w1 : Inport
  Constant : Constant  Value=RR
  Constant1 : Constant  Value=Lsig
  Constant2 : Constant  Value=V_base
  Constant3 : Constant  Value=w_base
  Divide : Product  Inputs=*/
  Max : MinMax  Function=max  Inputs=2
  Product : Product  Inputs=3
  Scope1 : Scope  NumInputPorts=2
  Scope2 : Scope  NumInputPorts=2
  Square : Math  Operator=square
  Kfw : Outport
  wires:
  Constant/1 -> Divide/1
  Constant1/1 -> Square/1
  Constant3/1 -> Scope1/1, Max/1
  w1/1 -> Scope1/2, Max/2
  Max/1 -> Product/3
  Constant2/1 -> Product/2
  Square/1 -> Product/1
  Product/1 -> Divide/2
  Divide/1 -> Scope2/1, Kfw/1

== system induction_foc/speed pi/Kis ==
  Id : Inport
  Constant : Constant
  Constant1 : Constant  Value=0.00001
  Divide : Product  Inputs=*/
  Gain : Gain  Gain=LM
  Gain1 : Gain  Gain=2*K^2*as^2*J/(3*np^2)
  Scope : Scope
  Scope1 : Scope
  Sum : Sum  Inputs=|++
  Kis : Outport
  wires:
  Id/1 -> Gain/1
  Gain/1 -> [psi]
  Divide/1 -> Scope1/1, Gain1/1
  Constant/1 -> Divide/1
  Gain1/1 -> Scope/1, Kis/1
  [psi] -> Sum/1
  Constant1/1 -> Sum/2
  Sum/1 -> Divide/2

== system induction_foc/speed pi/Kps1 ==
  Id : Inport
  Constant : Constant
  Divide : Product  Inputs=*/
  Gain : Gain  Gain=LM
  Gain1 : Gain  Gain=2*K^2*as*J/(3*np^2)
  Kps : Outport
  wires:
  Id/1 -> Gain/1
  Gain/1 -> [psi]
  Divide/1 -> Gain1/1
  Constant/1 -> Divide/1
  [psi] -> Divide/2
  Gain1/1 -> Kps/1

== system induction_foc/speed pi/Subsystem1 ==
  iq_ref_nonsat : Inport
  Add : Sum  Inputs=+-
  Constant : Constant  Value=2*I_base
  Gain : Gain  Gain=-1
  Max : MinMax  Function=max  Inputs=2
  Min : MinMax  Inputs=2
  Square Root : Sqrt
  Square1 : Math  Operator=square
  Square2 : Math  Operator=square
  iq_ref_sat : Outport
  wires:
  Gain/1 -> Max/2
  Min/1 -> Max/1
  Square2/1 -> Add/1
  iq_ref_nonsat/1 -> Min/1
  Constant/1 -> Square2/1
  Square1/1 -> Add/2
  Square Root/1 -> Gain/1, Min/2
  [Id_ref] -> Square1/1
  Add/1 -> Square Root/1
  Max/1 -> iq_ref_sat/1

== system induction_foc/speed pi/ba ==
  Id : Inport
  Constant : Constant
  Divide : Product  Inputs=*/
  Gain : Gain  Gain=LM
  Gain1 : Gain  Gain=2*K^2*as^2*J/(3*np^2)
  ba : Outport
  wires:
  Id/1 -> Gain/1
  Gain/1 -> [psi]
  Divide/1 -> Gain1/1
  Constant/1 -> Divide/1
  [psi] -> Divide/2
  Gain1/1 -> ba/1
